simulink model "PD_trajectory_controller_for_SOIPTD_parametric"  (R2019b)
settings: Solver=ode45  StartTime=0.0  StopTime=t_final  MaxStep=1e-3  RelTol=1e-3  EnableMultiTasking=on
undefined symbols (not defined in the file or in its folder): D, frequency, K, P, T1, T2, tau
libraries: simulink x1
settings Model: SimulationMode=accelerator  Creator=msa  LastModifiedBy=aaa_b
settings DataIOCC: SaveFormat=Array  DSMLogging=off  ReturnWorkspaceOutputs=off
settings OptimizationCC: LifeSpan=inf
settings DebuggingCC: SolverPrmCheckMsg=warning  SFUnexpectedBacktrackingDiag=warning  SFNoUnconditionalDefaultTransitionDiag=warning  SFExecutionAtInitializationDiag=none  ArithmeticOperatorsInVariantConditions=warning
settings HardwareCC: ProdBitPerPointer=32  ProdBitPerSizeT=32  ProdBitPerPtrDiffT=32  ProdLargestAtomicFloat=None  ProdIntDivRoundTo=Undefined  ProdEndianess=Unspecified  ProdWordSize=32  ProdHWDeviceType=32-bit Generic
settings ModelReferenceCC: PropagateSignalLabelsOutOfModel=off
settings SFSimCC: SimUseLocalCustomCode=off  CustomCodeUndefinedFunction=UseInterfaceOnly
settings RTWCC: RTWUseLocalCustomCode=off
settings CodeAppCC: StateflowObjectComments=on
settings GRTTargetCC: TargetLangStandard=C89/C90 (ANSI)  GeneratePreprocessorConditionals=Disable all
settings ConfigComp: CovMetricSettings=dw  CovHtmlReporting=on  CovSaveCumulativeToWorkspaceVar=on  CovSaveSingleToWorkspaceVar=on  CovExternalEMLEnable=off  CovSFcnEnable=off

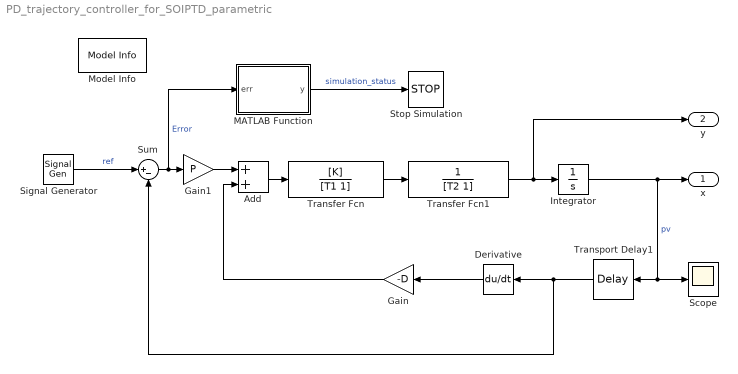
== system PD_trajectory_controller_for_SOIPTD_parametric ==
  Add : Sum
  Derivative : Derivative
  Gain : Gain  Gain=-D
  Gain1 : Gain  Gain=P
  Integrator : Integrator
  MATLAB Function : MATLAB Function  TreatAsAtomicUnit=on
  Model Info : simulink/Model-Wide Utilities/Model Info  Frame=on  DisplayStringWithTags=Model Info How should we take sensors reading WITHOUT delay  HorizontalTextAlignment=Center  LeftAlignmentValue=0.5
  Scope : Scope
  Signal Generator : SignalGenerator  Frequency=frequency  Units=rad/sec
  Stop Simulation : Stop
  Sum : Sum  Inputs=|+-
  Transfer Fcn : TransferFcn  Numerator=[K]  Denominator=[T1 1]
  Transfer Fcn1 : TransferFcn  Denominator=[T2 1]
  Transport Delay1 : TransportDelay  DelayTime=tau
  x : Outport  VectorParamsAs1DForOutWhenUnconnected=off
  y : Outport  Port=2  VectorParamsAs1DForOutWhenUnconnected=off
  wires:
  Transfer Fcn/1 -> Transfer Fcn1/1
  Transfer Fcn1/1 -> y/1, Integrator/1
  Add/1 -> Transfer Fcn/1
  Gain/1 -> Add/2
  Gain1/1 -> Add/1
  Sum/1 -> MATLAB Function/1(err), Gain1/1  "Error"
  Integrator/1 -> Scope/1, Transport Delay1/1, x/1  "pv"
  MATLAB Function/1(y) -> Stop Simulation/1  "simulation_status"
  Transport Delay1/1 -> Sum/2, Derivative/1
  Signal Generator/1 -> Sum/1  "ref"
  Derivative/1 -> Gain/1

== matlab function PD_trajectory_controller_for_SOIPTD_parametric/MATLAB Function ==
  data: err input; y output
function y = fcn(err)
if (abs(err)>1000)
    y=1;
else
    y=0;
end
